simulink model "ObservadorEE"  (Simulink 8.8)
settings: Solver=ode45  StartTime=0.0  StopTime=20  RelTol=1e-6  EnableMultiTasking=on
values from neighbouring files (symbols this model uses):
  K = acker(A,B,p)    [PrObsPertContinuoRed.m]    (also in PrPara2nl_PI.m = acker(Aa,Ba,[p,p,p]); TestesEE.m = acker(A,B,[p,p,p]); TestesEEcanalI.m = acker(A,B,[p,-.6-1.0198i,-.6+1.0198i]); TestesEEobsPert.m = acker(A,B,[p,-.6-1.0198i,-.6+1.0198i]))
  L = L'    [PrObsPertContinuoRed.m]    (also in PrPara2nl_PI.m; TestesEE.m; TestesEEcanalI.m; TestesEEobsPert.m)
  Nb = gf.den{1}(1,2)/gf.num{1}(1,2)    [PrObsPertContinuoRed.m]    (also in PrPara2nl_PI.m = gf.den{1}(1,3)/gf.num{1}(1,3); TestesEE.m = gf.den{1}(1,4)/gf.num{1}(1,4); TestesEEcanalI.m = gf.den{1}(1,4)/gf.num{1}(1,4); TestesEEobsPert.m = gf.den{1}(1,4)/gf.num{1}(1,4))
settings Model: SuppressorTable=22 serialization::archive 11 0 3 0 0 0 0 0  Creator=Adolfo  LastModifiedBy=adolfobs
settings OptimizationCC: ExpressionDepthLimit=2147483647  InitFltsAndDblsToZero=on
settings DebuggingCC: SaveWithParameterizedLinksMsg=none  SignalResolutionControl=TryResolveAllWithWarning  SolverPrmCheckMsg=warning  MultiTaskDSMMsg=warning  MultiTaskCondExecSysMsg=none
settings GRTTargetCC: TargetFcnLib=ansi_tfl_tmw.mat

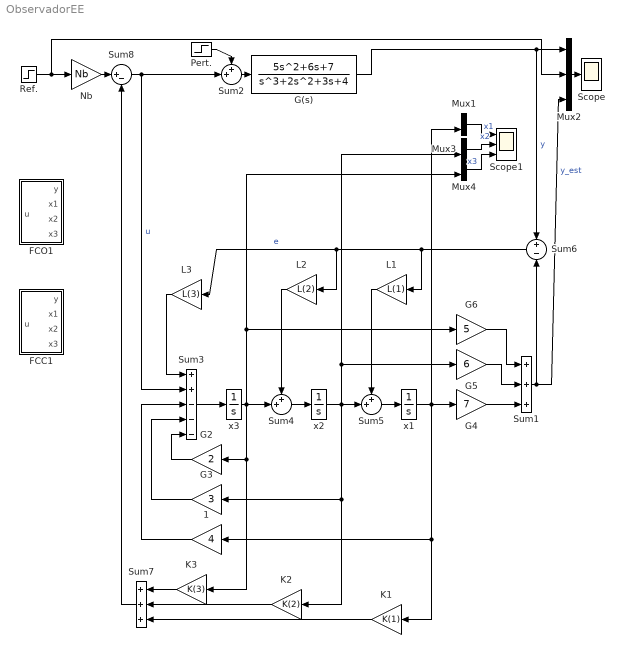
== system ObservadorEE ==
  1 : Gain  Gain=4
  FCC1 : Subsystem
  FCO1 : Subsystem
  G(s) : TransferFcn  Numerator=[5 6 7]  Denominator=[1 2 3 4]
  G2 : Gain  Gain=2
  G3 : Gain  Gain=3
  G4 : Gain  Gain=7
  G5 : Gain  Gain=6
  G6 : Gain  Gain=5
  K1 : Gain  Gain=K(1)
  K2 : Gain  Gain=K(2)
  K3 : Gain  Gain=K(3)
  L1 : Gain  Gain=L(1)
  L2 : Gain  Gain=L(2)
  L3 : Gain  Gain=L(3)
  Mux1 : Mux  Inputs=2
  Mux2 : Mux  Inputs=3
  Mux3 : Mux  Inputs=2
  Mux4 : Mux  Inputs=2
  Nb : Gain  Gain=Nb
  Pert. : Step  Time=10
  Ref. : Step  Time=5  SampleTime=0
  Scope : Scope
  Scope1 : Scope  NumInputPorts=3
  Sum1 : Sum  Inputs=+++
  Sum2 : Sum  Inputs=++|
  Sum3 : Sum  Inputs=++---
  Sum4 : Sum  Inputs=++|
  Sum5 : Sum  Inputs=++|
  Sum6 : Sum  Inputs=+-
  Sum7 : Sum  Inputs=+++
  Sum8 : Sum  Inputs=|+-
  x1 : Integrator  InitialCondition=3
  x2 : Integrator
  x3 : Integrator
  wires:
  Ref./1 -> Nb/1, Mux2/2
  Mux2/1 -> Scope/1
  x3/1 -> Sum4/2, G2/1, K3/1, G6/1, Mux4/2
  x2/1 -> Sum5/2, G3/1, K2/1, G5/1, Mux3/2
  Sum3/1 -> x3/1
  G2/1 -> Sum3/5
  G3/1 -> Sum3/4
  x1/1 -> Mux1/2, G4/1, 1/1, K1/1
  1/1 -> Sum3/3
  G4/1 -> Sum1/3
  G5/1 -> Sum1/2
  G6/1 -> Sum1/1
  Sum1/1 -> Sum6/2, Mux2/3  "y_est"
  Sum2/1 -> G(s)/1
  Sum4/1 -> x2/1
  Sum5/1 -> x1/1
  L3/1 -> Sum3/1
  L2/1 -> Sum4/1
  L1/1 -> Sum5/1
  K3/1 -> Sum7/1
  K2/1 -> Sum7/2
  K1/1 -> Sum7/3
  Sum8/1 -> Sum3/2, Sum2/2  "u"
  Nb/1 -> Sum8/1
  Sum6/1 -> L3/1, L2/1, L1/1  "e"
  Sum7/1 -> Sum8/2
  G(s)/1 -> Sum6/1, Mux2/1  "y"
  Mux1/1 -> Scope1/1  "x1"
  ? -> Mux1/1
  ? -> Mux3/1
  ? -> Mux4/1
  Mux4/1 -> Scope1/3  "x3"
  Mux3/1 -> Scope1/2  "x2"
  Pert./1 -> Sum2/1

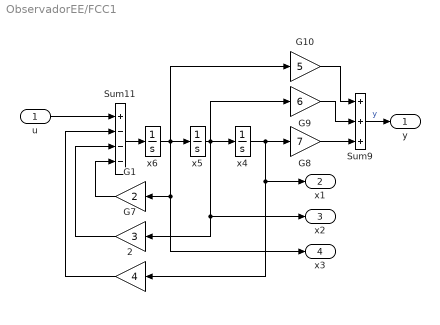
== system ObservadorEE/FCC1 ==
  u : Inport
  2 : Gain  Gain=4
  G1 : Gain  Gain=2
  G10 : Gain  Gain=5
  G7 : Gain  Gain=3
  G8 : Gain  Gain=7
  G9 : Gain  Gain=6
  Sum11 : Sum  Inputs=+---
  Sum9 : Sum  Inputs=+++
  x4 : Integrator
  x5 : Integrator
  x6 : Integrator  InitialCondition=1
  y : Outport
  x1 : Outport  Port=2
  x2 : Outport  Port=3
  x3 : Outport  Port=4
  wires:
  x6/1 -> G10/1, x5/1, G1/1, x3/1
  x5/1 -> G9/1, x4/1, G7/1, x2/1
  Sum11/1 -> x6/1
  G1/1 -> Sum11/4
  G7/1 -> Sum11/3
  x4/1 -> G8/1, 2/1, x1/1
  2/1 -> Sum11/2
  G8/1 -> Sum9/3
  G9/1 -> Sum9/2
  G10/1 -> Sum9/1
  u/1 -> Sum11/1
  Sum9/1 -> y/1  "y"

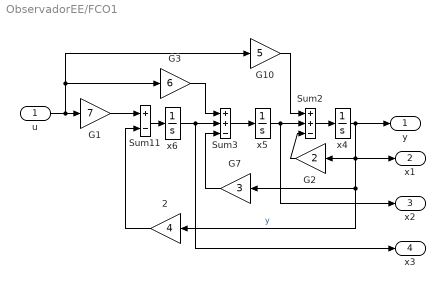
== system ObservadorEE/FCO1 ==
  u : Inport
  2 : Gain  Gain=4
  G1 : Gain  Gain=7
  G10 : Gain  Gain=5
  G2 : Gain  Gain=2
  G3 : Gain  Gain=6
  G7 : Gain  Gain=3
  Sum11 : Sum  Inputs=+-
  Sum2 : Sum  Inputs=++-
  Sum3 : Sum  Inputs=++-
  x4 : Integrator
  x5 : Integrator
  x6 : Integrator  InitialCondition=1
  y : Outport
  x1 : Outport  Port=2
  x2 : Outport  Port=3
  x3 : Outport  Port=4
  wires:
  x5/1 -> Sum2/2, x2/1
  Sum11/1 -> x6/1
  x4/1 -> x1/1, G2/1, 2/1, G7/1, y/1  "y"
  2/1 -> Sum11/2
  u/1 -> G1/1, G3/1, G10/1
  Sum2/1 -> x4/1
  G2/1 -> Sum2/3
  Sum3/1 -> x5/1
  G7/1 -> Sum3/3
  x6/1 -> Sum3/2, x3/1
  G1/1 -> Sum11/1
  G3/1 -> Sum3/1
  G10/1 -> Sum2/1
